simulink model "Smart_City_QCar2_VIRTUAL_car5"  (R2024b)
settings: Solver=ode1  StartTime=0.0  StopTime=inf  FixedStep=Controller_Sample_Time  RelTol=1e-3  EnableMultiTasking=on
values from neighbouring files (symbols this model uses):
  Audio_Sample_Time = 0.3    [Setup_QCar1and2_params.m]
  cameraStepSize = 3e-2    (= 0.03)    [Setup_QCar1and2_params.m]
  CSI_Sample_Time = 1/60    (= 0.0166666666667)    [Setup_QCar1and2_params.m]
  ImageDisplay_Sample_Time = CSI_Sample_Time*6    (= 0.1)    [Setup_QCar1and2_params.m]
  Initialization_Time = 5    [Setup_QCar1and2_params.m]
  LiDAR_Sample_Time = CSI_Sample_Time*3    (= 0.05)    [Setup_QCar1and2_params.m]
  map_mask = [1 1 1 0 0 1 0]    [Setup_QCar1and2_params.m]
  NN_Sample_Time = RealSense_Sample_Time*1    (= 0.0333333333333)    [Setup_QCar1and2_params.m]
  path_x = [0.826 0.836 0.846 0.856 0.866 0.876 0.886 0.896 0.906 0.916 0.926 0.936 ... (740 elements, 740x1)]    [SDCS_Paths_7.mat]
  path_x2 = [-0.614 -0.604 -0.594 -0.584 -0.574 -0.564 -0.554 -0.544 -0.534 -0.524 -0.514 -0.504 ... (1090 elements, 1090x1)]    [SDCS_Paths_7.mat]
  path_x3 = [-0.614 -0.603821428571 -0.593642857143 -0.583464285714 -0.573285714286 -0.563107142857 -0.552928571429 -0.54275 -0.532571428571 -0.522392857143 -0.512214285714 -0.502035714286 ... (714 elements, 714x1)]    [SDCS_Paths_7.mat]
  path_x4 = [-0.614 -0.604 -0.594 -0.584 -0.574 -0.564 -0.554 -0.544 -0.534 -0.524 -0.514 -0.504 ... (1761 elements, 1761x1)]    [SDCS_Paths_7.mat]
  path_x5 = [1.436 1.42588571429 1.41577142857 1.40565714286 1.39554285714 1.38542857143 1.37531428571 1.3652 1.35508571429 1.34497142857 1.33485714286 1.32474285714 ... (574 elements, 574x1)]    [SDCS_Paths_7.mat]
  path_x6 = [1.436 1.42588571429 1.41577142857 1.40565714286 1.39554285714 1.38542857143 1.37531428571 1.3652 1.35508571429 1.34497142857 1.33485714286 1.32474285714 ... (1288 elements, 1288x1)]    [SDCS_Paths_7.mat]
  path_x7 = [-1.5778487585 -1.56959877056 -1.56127865467 -1.55288878259 -1.54442952915 -1.53590127231 -1.52730439309 -1.51863927561 -1.50990630701 -1.50110587746 -1.49223838016 -1.4833042113 ... (2260 elements, 2260x1)]    [SDCS_Paths_7.mat]
  path_y = [-1.0887 -1.0887 -1.0887 -1.0887 -1.0887 -1.0887 -1.0887 -1.0887 -1.0887 -1.0887 -1.0887 -1.0887 ... (740 elements, 740x1)]    [SDCS_Paths_7.mat]
  path_y2 = [-1.0887 -1.0887 -1.0887 -1.0887 -1.0887 -1.0887 -1.0887 -1.0887 -1.0887 -1.0887 -1.0887 -1.0887 ... (1090 elements, 1090x1)]    [SDCS_Paths_7.mat]
  path_y3 = [-1.0887 -1.0887 -1.0887 -1.0887 -1.0887 -1.0887 -1.0887 -1.0887 -1.0887 -1.0887 -1.0887 -1.0887 ... (714 elements, 714x1)]    [SDCS_Paths_7.mat]
  path_y4 = [-1.0887 -1.0887 -1.0887 -1.0887 -1.0887 -1.0887 -1.0887 -1.0887 -1.0887 -1.0887 -1.0887 -1.0887 ... (1761 elements, 1761x1)]    [SDCS_Paths_7.mat]
  path_y5 = [-0.8157 -0.8157 -0.8157 -0.8157 -0.8157 -0.8157 -0.8157 -0.8157 -0.8157 -0.8157 -0.8157 -0.8157 ... (574 elements, 574x1)]    [SDCS_Paths_7.mat]
  path_y6 = [-0.8157 -0.8157 -0.8157 -0.8157 -0.8157 -0.8157 -0.8157 -0.8157 -0.8157 -0.8157 -0.8157 -0.8157 ... (1288 elements, 1288x1)]    [SDCS_Paths_7.mat]
  path_y7 = [-0.614490295955 -0.61974988896 -0.624981792226 -0.630185771997 -0.635361595765 -0.640509032279 -0.645627851559 -0.6507178249 -0.655778724888 -0.660810325409 -0.665812401655 -0.670784730139 ... (2260 elements, 2260x1)]    [SDCS_Paths_7.mat]
  RealSense_Sample_Time = CSI_Sample_Time*2    (= 0.0333333333333)    [Setup_QCar1and2_params.m]
undefined symbols (not defined in the file or in its folder): DiscIntNeverNeededParam, gcbh, Joystick_Sample_Time, JPEG, qc_get_step_size, video_display_show
libraries: quarc_library x61, simulink_extras x9, simulink x5
(part 2 of 4)

== system Smart_City_QCar2_VIRTUAL_car5/Rate Timing Plots/monitorTiming7 ==
  note: Timing Performance
  note: moniorTiming Module:
      |
      | This subsystem outputs the sample time and computation time of the model.
      |
      | Outputs:
      | sampleTime (s) n/a : Sample time (unfiltered and filtered) in seconds.
      | computationTime (s) n/a : Computation time (unfiltered and filtered) in seconds.
      |
      | Usage:
      | Compare the Sample Time (s) output to a constant (qc_get_step_size) to monitor whether or not the desired sample time is being achieved. The Computation Time (s) values should be lower than the corresponding sample time value to ensure that the solver has enough time per time step.
  Computation Time : quarc_library/Sources/Time/Computation Time  sample_time=1  use_model=on  use_cpu_time=off
  Constant : Constant  SampleTime=-1
  Mux : Mux  Inputs=3
  Sample Time : quarc_library/Sources/Time/Sample Time  Priority=-99  sample_time=1
  Timing (s) : Outport  VectorParamsAs1DForOutWhenUnconnected=off
  wires:
  Computation Time/1 -> Mux/3
  Mux/1 -> Timing (s)/1
  Sample Time/1 -> Mux/1
  Constant/1 -> Mux/2

== system Smart_City_QCar2_VIRTUAL_car5/Rate Timing Plots/monitorTiming8 ==
  note: moniorTiming Module:
      |
      | This subsystem outputs the sample time and computation time of the model.
      |
      | Outputs:
      | sampleTime (s) n/a : Sample time (unfiltered and filtered) in seconds.
      | computationTime (s) n/a : Computation time (unfiltered and filtered) in seconds.
      |
      | Usage:
      | Compare the Sample Time (s) output to a constant (qc_get_step_size) to monitor whether or not the desired sample time is being achieved. The Computation Time (s) values should be lower than the corresponding sample time value to ensure that the solver has enough time per time step.
  note: Timing Performance
  Computation Time : quarc_library/Sources/Time/Computation Time  sample_time=Audio_Sample_Time  use_model=on  use_cpu_time=off
  Constant : Constant  Value=Audio_Sample_Time  SampleTime=-1
  Mux : Mux  Inputs=3
  Sample Time : quarc_library/Sources/Time/Sample Time  Priority=-99  sample_time=Audio_Sample_Time
  Timing (s) : Outport  VectorParamsAs1DForOutWhenUnconnected=off
  wires:
  Constant/1 -> Mux/2
  Sample Time/1 -> Mux/1
  Mux/1 -> Timing (s)/1
  Computation Time/1 -> Mux/3

== system Smart_City_QCar2_VIRTUAL_car5/RealSense Camera/Newer Depth ==
  In1 : Inport
  Channel : quarc_library/Signal Routing/Channel  channel=0  buffer_size=1
  Image Compress : quarc_library/Image Processing/Generic/Image Compress  algorithm=JPEG  source=Internal dialog parameter  quality=quality  output_dim=-1
  Video Display : quarc_library/Multimedia/Video Display  Tag=Smart_City_QCar2_VIRTUAL_car5/RealSense Camera/Newer Depth/Video Display  sample_time=sample_time  use_hardware=on
  wires:
  Image Compress/1 -> Channel/1
  In1/1 -> Image Compress/1
  Channel/1 -> Video Display/1

== system Smart_City_QCar2_VIRTUAL_car5/RealSense Camera/obstacleDetection Markham March 22 ==
  note: This function looks within the area of interest and finds the 25% smallest point to use as the distance
  note: m
  note: %
  note: %
  note: px
  note: px
  note: %
  note: m
  note: %
  imageDepth : Inport
  steering (rad) : Inport  Port=2
  new_depth : EnablePort  PropagateVarSize=During execution
  Add : Sum
  Bias : Constant  Value=0
  Box Color : Constant  Value=[255 0 0]
  Constant1 : Constant  Value=200
  Constant2 : Constant  Value=0.1
  Constant3 : Constant  Value=5
  Constant4 : Constant  Value=50
  Constant5 : Constant  Value=.55
  Constant6 : Constant  Value=0.5
  Constant7 : Constant  Value=0.5
  Constant8 : Constant
  Draw Lines Module : MATLAB Function  TreatAsAtomicUnit=on
  Saturation : Saturate  UpperLimit=10  LowerLimit=0.05
  Steering based image subselector : MATLAB Function  TreatAsAtomicUnit=on
  Terminator{,1..6} (7 alike) : Terminator
  imageDepthForDisplay : Outport  VectorParamsAs1DForOutWhenUnconnected=off
  distance (m) : Outport  Port=2
  wires:
  Draw Lines Module/1(img_out) -> imageDepthForDisplay/1
  Box Color/1 -> Draw Lines Module/3(color)
  Constant2/1 -> Steering based image subselector/3(minDistance)
  Constant4/1 -> Steering based image subselector/6(height)
  Steering based image subselector/1(pts) -> Draw Lines Module/2(pts)
  Constant8/1 -> Steering based image subselector/10(maxSteeringWidth)
  Constant7/1 -> Steering based image subselector/9(reduction)
  Constant1/1 -> Steering based image subselector/5(width)
  Constant5/1 -> Steering based image subselector/7(vertCenter)
  Constant6/1 -> Steering based image subselector/8(maxSteering)
  Constant3/1 -> Steering based image subselector/4(maxDistance)
  Saturation/1 -> distance (m)/1
  Bias/1 -> Add/2
  Add/1 -> Saturation/1
  Steering based image subselector/8(pt_25) -> Add/1
  imageDepth/1 -> Steering based image subselector/1(depth), Draw Lines Module/1(img_in)
  steering (rad)/1 -> Steering based image subselector/2(steering)
  Steering based image subselector/2(distance) -> Terminator/1
  Steering based image subselector/3(median_pts) -> Terminator1/1
  Steering based image subselector/4(mean_pts) -> Terminator2/1
  Steering based image subselector/5(min_pts) -> Terminator3/1
  Steering based image subselector/6(max_pts) -> Terminator4/1
  Steering based image subselector/7(num_pts) -> Terminator5/1
  Steering based image subselector/9(mean_middle) -> Terminator6/1

== system Smart_City_QCar2_VIRTUAL_car5/Speed & Steering Commander/Cross Track Controller ==
  closest point : Inport
  distance : Inport  Port=2
  xy : Inport  Port=3
  Heading : Inport  Port=4
  Commanded_Speed : Inport  Port=5
  Path : Inport  Port=6
  Constant : Constant  Value=0
  Constant1 : Constant
  Constant6 : Constant  Value=Initialization_Time
  Cos : Trigonometry  Operator=cos
  Cos1 : Trigonometry
  Cross Product : quarc_library/Math Operations/Vectors/Cross Product
      settings: SourceProductName=QUARC Targets
  Demux : Demux  Outputs=3
  Equal : RelationalOperator  Operator===  OutDataTypeStr=boolean  RndMeth=Simplest  InputSameDT=off
  Equal1 : RelationalOperator  Operator=~=  OutDataTypeStr=boolean  RndMeth=Simplest  InputSameDT=off
  Gain3 : Gain
  Gain6 : Gain  Gain=3
  GreaterThan : RelationalOperator  Operator=<  OutDataTypeStr=boolean  RndMeth=Simplest  InputSameDT=off
  Integrator : Integrator  ExternalReset=level  LimitOutput=on  UpperSaturationLimit=.2  LowerSaturationLimit=-.2
  Integrator1 : Integrator  ExternalReset=level  LimitOutput=on  UpperSaturationLimit=1  LowerSaturationLimit=0
  Memory1 : Memory  InitialCondition=6  InheritSampleTime=on  LinearizeMemory=on  LinearizeAsDelay=on
  Mux : Mux  Inputs=3
  Mux1 : Mux  Inputs=2
  Mux2 : Mux  Inputs=2
  OR : Logic  Operator=OR  Inputs=3  IconShape=distinctive  AllPortsSameDT=off  OutDataTypeStr=boolean
  Product : Product
  Product3 : Product
  Radians to Degrees : simulink_extras/Transformations/Radians to Degrees
  Saturation1 : Saturate  UpperLimit=.2  LowerLimit=-.2
  Scope1 : Scope  NumInputPorts=2
  Sign : Signum
  Sum : Sum  Inputs=+-
  Sum2 : Sum
  Time1 : quarc_library/Sources/Time/Time  time_source=Wall clock  sample_time=qc_get_step_size
  steering correction : Outport
  wires:
  Heading/1 -> Cos1/1, Cos/1
  Cos/1 -> Mux/1
  Cos1/1 -> Mux/2
  xy/1 -> Sum/2
  closest point/1 -> Sum/1
  Sum/1 -> Mux1/1
  Mux1/1 -> Cross Product/2
  Mux/1 -> Cross Product/1
  Cross Product/1 -> Demux/1
  Demux/3 -> Sign/1
  Sign/1 -> Product3/1
  Gain6/1 -> Integrator/1
  Product3/1 -> Gain3/1, Gain6/1
  Integrator/1 -> Mux2/1, Sum2/1
  Saturation1/1 -> Mux2/2, Sum2/2
  distance/1 -> Product3/2
  Sum2/1 -> steering correction/1
  Commanded_Speed/1 -> Equal/1
  Constant/1 -> Equal/2
  Path/1 -> Equal1/2, Memory1/1
  Memory1/1 -> Equal1/1
  Equal1/1 -> OR/2
  Equal/1 -> OR/1
  OR/1 -> Scope1/1, Integrator1/2, Integrator/2
  Constant1/1 -> Integrator1/1
  Product/1 -> Saturation1/1
  Gain3/1 -> Product/1
  Integrator1/1 -> Product/2
  Mux2/1 -> Radians to Degrees/1
  Radians to Degrees/1 -> Scope1/2
  Time1/1 -> GreaterThan/1
  Constant6/1 -> GreaterThan/2
  GreaterThan/1 -> OR/3

== system Smart_City_QCar2_VIRTUAL_car5/Speed & Steering Commander/Infrastructure Car Detection Speed Adjust ==
  obstacleDistance (m) : Inport
  Desired Speed Command : Inport  Port=2
  Constant : Constant  Value=0.3
  Constant1 : Constant  Value=.4
  Constant2 : Constant
  Less Than : RelationalOperator  Operator=<  OutDataTypeStr=boolean  RndMeth=Simplest  InputSameDT=off
  MATLAB Function : MATLAB Function  TreatAsAtomicUnit=on
  Scope : Scope  NumInputPorts=2
  Adjusted Speed Command : Outport  VectorParamsAs1DForOutWhenUnconnected=off
  Honk : Outport  Port=2
  wires:
  Desired Speed Command/1 -> MATLAB Function/4(nominal_speed)
  MATLAB Function/1(speed_cmd) -> Adjusted Speed Command/1, Scope/1
  Less Than/1 -> Honk/1
  Constant1/1 -> Less Than/2
  obstacleDistance (m)/1 -> MATLAB Function/1(obstacle_distance), Scope/2, Less Than/1
  Constant/1 -> MATLAB Function/2(stop_distance)  "stop distance (m)"
  Constant2/1 -> MATLAB Function/3(nominal_tracking_distance)  "nominal tracking distance (m)"

== system Smart_City_QCar2_VIRTUAL_car5/Speed & Steering Commander/Path Commander ==
  note: Tunable
      | Params
  note: Changed the abs and the duration
  path : Inport
  xy : Inport  Port=2
  look_ahead_d : Inport  Port=3
  Data Type Conversion : DataTypeConversion  SaturateOnIntegerOverflow=off  RndMeth=Floor
  Display : Display
  "Distance  " : Scope
  Distance (m) to a viable path : Constant  Value=0.05
  Duration that car is within distance of viable path : Constant  Value=0.35
  Less Than Threshold : Subsystem
  Multiport Switch : MultiPortSwitch  Inputs=7  DiagnosticForDefault=None  SaturateOnIntegerOverflow=off  InputSameDT=off
  Multiport Switch1 : MultiPortSwitch  Inputs=7  DiagnosticForDefault=None  SaturateOnIntegerOverflow=off  InputSameDT=off
  Multiport Switch2 : MultiPortSwitch  Inputs=7  DiagnosticForDefault=None  SaturateOnIntegerOverflow=off  InputSameDT=off
  Mux : Mux  Inputs=7
  Path 1  Look Ahead Generator : Subsystem
  Path 2  Look Ahead Generator : Subsystem
  Path 3  Look Ahead Generator : Subsystem
  Path 4  Look Ahead Generator : Subsystem
  Path 5  Look Ahead Generator : Subsystem
  Path 6  Look Ahead Generator : Subsystem
  Path 7  Look Ahead Generator : Subsystem
  Turn Paths on and Off : Gain  Gain=map_mask
  xy_cmd : Outport
  Path_Options : Outport  Port=2
  closest point : Outport  Port=3
  distance : Outport  Port=4
  wires:
  look_ahead_d/1 -> Path 7  Look Ahead Generator/2(look_ahead_d), Path 6  Look Ahead Generator/2(look_ahead_d), Path 5  Look Ahead Generator/2(look_ahead_d), Path 4  Look Ahead Generator/2(look_ahead_d), Path 3  Look Ahead Generator/2(look_ahead_d), Path 2  Look Ahead Generator/2(look_ahead_d), Path 1  Look Ahead Generator/2(look_ahead_d)
  path/1 -> Multiport Switch2/1, Multiport Switch1/1, Multiport Switch/1
  Path 1  Look Ahead Generator/1(xy_cmd) -> Multiport Switch/2
  Path 2  Look Ahead Generator/1(xy_cmd) -> Multiport Switch/3
  Multiport Switch/1 -> xy_cmd/1
  Path 3  Look Ahead Generator/1(xy_cmd) -> Multiport Switch/4
  Path 4  Look Ahead Generator/1(xy_cmd) -> Multiport Switch/5
  Path 1  Look Ahead Generator/3(distance) -> Multiport Switch2/2, Mux/1
  Path 2  Look Ahead Generator/3(distance) -> Multiport Switch2/3, Mux/2
  Path 3  Look Ahead Generator/3(distance) -> Multiport Switch2/4, Mux/3
  Path 4  Look Ahead Generator/3(distance) -> Multiport Switch2/5, Mux/4
  Mux/1 -> "Distance  "/1, Less Than Threshold/1(Distances)
  Distance (m) to a viable path/1 -> Less Than Threshold/2(Distance Threshold)
  Duration that car is within distance of viable path/1 -> Less Than Threshold/3(Duration Threshold)
  Less Than Threshold/1(elapsed) -> Data Type Conversion/1, Display/1
  Turn Paths on and Off/1 -> Path_Options/1
  Data Type Conversion/1 -> Turn Paths on and Off/1
  Path 5  Look Ahead Generator/1(xy_cmd) -> Multiport Switch/6
  Path 6  Look Ahead Generator/1(xy_cmd) -> Multiport Switch/7
  Path 5  Look Ahead Generator/3(distance) -> Multiport Switch2/6, Mux/5
  Path 6  Look Ahead Generator/3(distance) -> Multiport Switch2/7, Mux/6
  Path 1  Look Ahead Generator/2(closest_point) -> Multiport Switch1/2
  Path 2  Look Ahead Generator/2(closest_point) -> Multiport Switch1/3
  Path 3  Look Ahead Generator/2(closest_point) -> Multiport Switch1/4
  Path 4  Look Ahead Generator/2(closest_point) -> Multiport Switch1/5
  Path 5  Look Ahead Generator/2(closest_point) -> Multiport Switch1/6
  Path 6  Look Ahead Generator/2(closest_point) -> Multiport Switch1/7
  Multiport Switch1/1 -> closest point/1
  Multiport Switch2/1 -> distance/1
  xy/1 -> Path 7  Look Ahead Generator/1(xy), Path 6  Look Ahead Generator/1(xy), Path 5  Look Ahead Generator/1(xy), Path 4  Look Ahead Generator/1(xy), Path 3  Look Ahead Generator/1(xy), Path 2  Look Ahead Generator/1(xy), Path 1  Look Ahead Generator/1(xy)
  Path 7  Look Ahead Generator/1(xy_cmd) -> Multiport Switch/8
  Path 7  Look Ahead Generator/2(closest_point) -> Multiport Switch1/8
  Path 7  Look Ahead Generator/3(distance) -> Mux/7, Multiport Switch2/8

== system Smart_City_QCar2_VIRTUAL_car5/Speed & Steering Commander/Realsense Obstacle Detection Speed Adjust ==
  obstacleDistance (m) : Inport
  Desired Speed Command : Inport  Port=2
  Constant : Constant  Value=0.5
  Constant1 : Constant  Value=0.5
  Constant2 : Constant  Value=0.75
  Less Than : RelationalOperator  Operator=<  OutDataTypeStr=boolean  RndMeth=Simplest  InputSameDT=off
  MATLAB Function : MATLAB Function  TreatAsAtomicUnit=on
  Scope : Scope  NumInputPorts=2
  Adjusted Speed Command : Outport  VectorParamsAs1DForOutWhenUnconnected=off
  Honk : Outport  Port=2
  wires:
  Constant2/1 -> MATLAB Function/3(nominal_tracking_distance)  "nominal tracking distance (m)"
  Constant/1 -> MATLAB Function/2(stop_distance)  "stop distance (m)"
  obstacleDistance (m)/1 -> Less Than/1, Scope/2, MATLAB Function/1(obstacle_distance)
  Constant1/1 -> Less Than/2
  Less Than/1 -> Honk/1
  MATLAB Function/1(speed_cmd) -> Scope/1, Adjusted Speed Command/1
  Desired Speed Command/1 -> MATLAB Function/4(nominal_speed)

== system Smart_City_QCar2_VIRTUAL_car5/Speed & Steering Commander/Steering Based on LiDAR ==
  xy_command : Inport
  xy : Inport  Port=2
  heading : Inport  Port=3
  Direction Vector Generator : Subsystem
  Display1 : Display
      settings: Decimation=100
  Gain1 : Gain
  Radians to Degrees1 : simulink_extras/Transformations/Radians to Degrees
  Steering Commander : MATLAB Function  TreatAsAtomicUnit=on
  distance : Outport
  LiDAR Steering : Outport  Port=2
  wires:
  Direction Vector Generator/1(distance) -> distance/1
  xy_command/1 -> Direction Vector Generator/1(xy_command)
  Direction Vector Generator/2(aoa) -> Radians to Degrees1/1, Steering Commander/1(aoa)
  Gain1/1 -> LiDAR Steering/1
  Radians to Degrees1/1 -> Display1/1
  xy/1 -> Direction Vector Generator/2(xy)
  heading/1 -> Direction Vector Generator/3(heading)
  Steering Commander/1(steering) -> Gain1/1

== system Smart_City_QCar2_VIRTUAL_car5/Speed & Steering Commander/Traffic Zone 1 ==
  note: [1 -.3] %[1,5 0]
  note: [0.2 -0.7]
  note: select the control variable
  xy : Inport
  speed in : Inport  Port=2
  Traffic Light : Inport  Port=3
  AND : Logic  Inputs=4  IconShape=distinctive  AllPortsSameDT=off  OutDataTypeStr=boolean
  Bias : Bias  SaturateOnIntegerOverflow=off
  Constant13 : Constant  Value=[-0.61 -1.21]
  Constant14 : Constant  Value=[0 -0.86]
  Constant3 : Constant  Value=.1
  Demux : Demux  Outputs=2
  Demux1 : Demux  Outputs=2
  Demux2 : Demux  Outputs=2
  Display : Display
  Gain : Gain  Gain=-1
  Greater Than Threshold : Subsystem
  Less Than Threshold : Subsystem
  MATLAB Function2 : MATLAB Function  TreatAsAtomicUnit=on
  Memory7 : Memory  InitialCondition=1  InheritSampleTime=on  LinearizeMemory=on  LinearizeAsDelay=on
  Saturation : Saturate  UpperLimit=1  LowerLimit=0
  "Speed " : Scope
  Speed Multi : Scope
  Traffic State : Display
  in zone : Display
  Speed Out : Outport
  wires:
  xy/1 -> Greater Than Threshold/1(Signal), Less Than Threshold/1(Signal), Demux2/1
  Constant3/1 -> Less Than Threshold/3(Duration), Greater Than Threshold/3(Duration)
  Constant13/1 -> Greater Than Threshold/2(Threshold)
  Constant14/1 -> Less Than Threshold/2(Threshold)
  Greater Than Threshold/1(elapsed) -> Demux/1
  Demux/2 -> AND/2
  Demux/1 -> AND/1
  Less Than Threshold/1(elapsed) -> Demux1/1
  Demux1/2 -> AND/4
  Demux1/1 -> AND/3
  Demux2/1 -> Bias/1
  Bias/1 -> Gain/1
  Gain/1 -> Saturation/1
  MATLAB Function2/1(Traffic_State) -> Memory7/1, Traffic State/1
  Memory7/1 -> MATLAB Function2/1(Previous_State)
  speed in/1 -> MATLAB Function2/2(Speed_In)
  AND/1 -> MATLAB Function2/4(In_Zone), in zone/1
  Saturation/1 -> Speed Multi/1, MATLAB Function2/3(Speed_Multi)
  MATLAB Function2/2(Speed_Out) -> Speed Out/1, "Speed "/1
  Traffic Light/1 -> Display/1, MATLAB Function2/5(Traffic_Light)  "1 means green"

== system Smart_City_QCar2_VIRTUAL_car5/Speed & Steering Commander/Traffic Zone 2 ==
  note: select the control variable
  xy : Inport
  speed in : Inport  Port=2
  Traffic Light : Inport  Port=3
  AND : Logic  Inputs=4  IconShape=distinctive  AllPortsSameDT=off  OutDataTypeStr=boolean
  Bias : Bias  Bias=-0.8  SaturateOnIntegerOverflow=off
  Constant13 : Constant  Value=[0.75 -0.9]
  Constant14 : Constant  Value=[1.35 -0.65]
  Constant3 : Constant  Value=.1
  Demux : Demux  Outputs=2
  Demux1 : Demux  Outputs=2
  Demux2 : Demux  Outputs=2
  Display : Display
  Gain : Gain
  Greater Than Threshold : Subsystem
  Less Than Threshold : Subsystem
  MATLAB Function2 : MATLAB Function  TreatAsAtomicUnit=on
  Memory7 : Memory  InitialCondition=1  InheritSampleTime=on  LinearizeMemory=on  LinearizeAsDelay=on
  Saturation : Saturate  UpperLimit=1  LowerLimit=0
  "Speed " : Scope
  Speed Multi : Scope
  Traffic State : Display
  in zone : Display
  Speed Out : Outport
  wires:
  MATLAB Function2/2(Speed_Out) -> "Speed "/1, Speed Out/1
  Saturation/1 -> MATLAB Function2/3(Speed_Multi), Speed Multi/1
  AND/1 -> in zone/1, MATLAB Function2/4(In_Zone)
  speed in/1 -> MATLAB Function2/2(Speed_In)
  Memory7/1 -> MATLAB Function2/1(Previous_State)
  MATLAB Function2/1(Traffic_State) -> Traffic State/1, Memory7/1
  Gain/1 -> Saturation/1
  Bias/1 -> Gain/1
  Demux2/1 -> Bias/1
  Demux1/1 -> AND/3
  Demux1/2 -> AND/4
  Less Than Threshold/1(elapsed) -> Demux1/1
  Demux/1 -> AND/1
  Demux/2 -> AND/2
  Greater Than Threshold/1(elapsed) -> Demux/1
  Constant14/1 -> Less Than Threshold/2(Threshold)
  Constant13/1 -> Greater Than Threshold/2(Threshold)
  Constant3/1 -> Greater Than Threshold/3(Duration), Less Than Threshold/3(Duration)
  xy/1 -> Greater Than Threshold/1(Signal), Less Than Threshold/1(Signal), Demux2/1
  Traffic Light/1 -> Display/1, MATLAB Function2/5(Traffic_Light)

== system Smart_City_QCar2_VIRTUAL_car5/Speed & Steering Commander/xy signal maker ==
  xy 1 : Inport
  xy 2 : Inport  Port=2
  Demux1 : Demux  Outputs=2
  Demux2 : Demux  Outputs=2
  Mux : Mux  Inputs=2
  Mux1 : Mux  Inputs=2
  Rate Transition1 : RateTransition  OutPortSampleTime=ImageDisplay_Sample_Time
  Rate Transition2 : RateTransition  OutPortSampleTime=ImageDisplay_Sample_Time
  x : Outport
  y : Outport  Port=2
  wires:
  Demux2/1 -> Mux/2
  Demux1/2 -> Mux1/1
  Demux1/1 -> Mux/1
  Demux2/2 -> Mux1/2
  Mux/1 -> x/1
  Mux1/1 -> y/1
  xy 1/1 -> Rate Transition1/1
  Rate Transition1/1 -> Demux1/1
  xy 2/1 -> Rate Transition2/1
  Rate Transition2/1 -> Demux2/1

== system Smart_City_QCar2_VIRTUAL_car5/QCar/To//From Simulation/RGB ==
  In1 : Inport
  Enable : EnablePort  StatesWhenEnabling=reset
  Image Decompress : quarc_library/Image Processing/Generic/Image Decompress  algorithm=JPEG  resolution=custom  width=820  height=410  output_format=MATLAB RGB (HxWx3)  data_type=uint8
      settings: AttributesFormatString=(%<algorithm>)  SourceProductName=QUARC Targets
  RGB : Outport  VectorParamsAs1DForOutWhenUnconnected=off
  wires:
  Image Decompress/1 -> RGB/1
  In1/1 -> Image Decompress/1

== system Smart_City_QCar2_VIRTUAL_car5/QCar/To//From Simulation/RGB1 ==
  In1 : Inport
  Enable : EnablePort  StatesWhenEnabling=reset
  Image Decompress : quarc_library/Image Processing/Generic/Image Decompress  algorithm=JPEG  resolution=custom  width=820  height=410  output_format=MATLAB RGB (HxWx3)  data_type=uint8
      settings: AttributesFormatString=(%<algorithm>)  SourceProductName=QUARC Targets
  RGB : Outport  VectorParamsAs1DForOutWhenUnconnected=off
  wires:
  Image Decompress/1 -> RGB/1
  In1/1 -> Image Decompress/1

== system Smart_City_QCar2_VIRTUAL_car5/QCar/To//From Simulation/RGB2 ==
  In1 : Inport
  Enable : EnablePort  StatesWhenEnabling=reset
  Image Decompress : quarc_library/Image Processing/Generic/Image Decompress  algorithm=JPEG  resolution=custom  width=820  height=410  output_format=MATLAB RGB (HxWx3)  data_type=uint8
      settings: AttributesFormatString=(%<algorithm>)  SourceProductName=QUARC Targets
  RGB : Outport  VectorParamsAs1DForOutWhenUnconnected=off
  wires:
  Image Decompress/1 -> RGB/1
  In1/1 -> Image Decompress/1

== system Smart_City_QCar2_VIRTUAL_car5/QCar/To//From Simulation/RGB3 ==
  In1 : Inport
  Enable : EnablePort  StatesWhenEnabling=reset
  Image Decompress : quarc_library/Image Processing/Generic/Image Decompress  algorithm=JPEG  resolution=custom  width=820  height=410  output_format=MATLAB RGB (HxWx3)  data_type=uint8
      settings: AttributesFormatString=(%<algorithm>)  SourceProductName=QUARC Targets
  RGB : Outport  VectorParamsAs1DForOutWhenUnconnected=off
  wires:
  Image Decompress/1 -> RGB/1
  In1/1 -> Image Decompress/1

== system Smart_City_QCar2_VIRTUAL_car5/QCar/To//From Simulation/RGB4 ==
  In1 : Inport
  Enable : EnablePort  StatesWhenEnabling=reset
  Image Decompress : quarc_library/Image Processing/Generic/Image Decompress  algorithm=JPEG  resolution=640 x 480  width=640  height=480  output_format=MATLAB RGB (HxWx3)  data_type=uint8
      settings: AttributesFormatString=(%<algorithm>)  SourceProductName=QUARC Targets
  RGB : Outport  VectorParamsAs1DForOutWhenUnconnected=off
  wires:
  Image Decompress/1 -> RGB/1
  In1/1 -> Image Decompress/1

== system Smart_City_QCar2_VIRTUAL_car5/QCar/To//From Simulation/RGB5 ==
  In1 : Inport
  Enable : EnablePort  StatesWhenEnabling=reset
  Image Decompress : quarc_library/Image Processing/Generic/Image Decompress  algorithm=JPEG  resolution=640 x 480  width=640  height=480  output_format=MATLAB greyscale (HxW)  data_type=uint8
      settings: AttributesFormatString=(%<algorithm>)  SourceProductName=QUARC Targets
  RGB : Outport  VectorParamsAs1DForOutWhenUnconnected=off
  wires:
  Image Decompress/1 -> RGB/1
  In1/1 -> Image Decompress/1

== system Smart_City_QCar2_VIRTUAL_car5/QCar/To//From Simulation/Subsystem ==
  dist : Inport
  angles : Inport  Port=2
  Gain : Gain  Gain=0.1
  Polar Figure : quarc_library/Sinks/Figures/Polar Figure  figure_mode=Use figure window  figure_tag=figure1  axes_tag=axes1  plot_mode=Frame-based  minimum_rho=0  maximum_rho=2  minimum_theta=0  maximum_theta=360  zero_location=top  direction=counterclockwise  buffer_size=1  update_rate=100  sample_time=-1  initial_position="2561      343.66667           1920      983.33333"  initial_visibility=off  line1_style=Solid line (-)  line1_width=0.5  line1_color=[0 0.4470 0.7410]  marker1=Circle (o)  marker1_size=2  marker1_edge_color=[0 0.447059 0.741176]  marker1_face_color=[0 0.447059 0.741176]  line2_style=Solid line (-)  line2_width=0.5  line2_color=[0.85098 0.32549 0.0980392]  marker2=None  marker2_size=6  marker2_edge_color=[0.85098 0.32549 0.0980392]  marker2_face_color=[0.85098 0.32549 0.0980392]  line3_style=Solid line (-)  line3_width=0.5  line3_color=[0.929412 0.694118 0.12549]  marker3=None  marker3_size=6  marker3_edge_color=[0.929412 0.694118 0.12549]  marker3_face_color=[0.929412 0.694118 0.12549]  line4_style=Solid line (-)  line4_width=0.5  line4_color=[0.494118 0.184314 0.556863]  marker4=None  marker4_size=6  marker4_edge_color=[0.494118 0.184314 0.556863]  marker4_face_color=[0.494118 0.184314 0.556863]  line5_style=Solid line (-)  line5_width=0.5  line5_color=[0.466667 0.67451 0.188235]  marker5=None  marker5_size=6  marker5_edge_color=[0.466667 0.67451 0.188235]  marker5_face_color=[0.466667 0.67451 0.188235]
      settings: SourceProductName=QUARC Targets
  wires:
  Gain/1 -> Polar Figure/1
  dist/1 -> Gain/1
  angles/1 -> Polar Figure/2

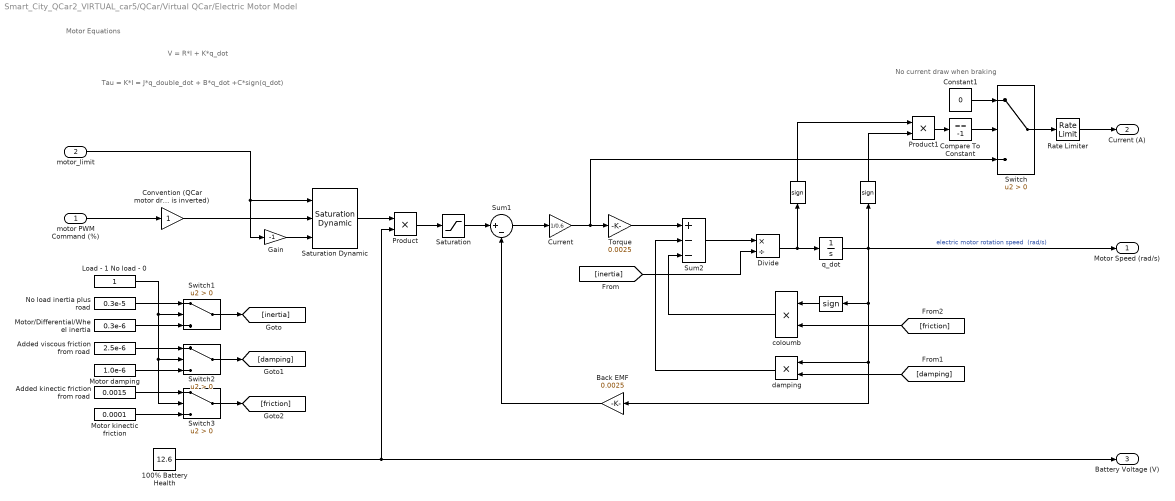
== system Smart_City_QCar2_VIRTUAL_car5/QCar/Virtual QCar/Electric Motor Model ==
  note: No current draw when braking
  note: Motor Equations
  note: Tau = K*I = J*q_double_dot + B*q_dot +C*sign(q_dot)
  note: V = R*I + K*q_dot
  motor PWM Command (%) : Inport
  motor_limit : Inport  Port=2
  " " : Signum
  "  " : Signum
  "   " : Signum
  100% Battery Health : Constant  Value=12.6
  Added kinectic friction from road : Constant  Value=0.0015
  Added viscous friction from road : Constant  Value=2.5e-6
  Back EMF : Gain  Gain=0.0025
  Compare To Constant : simulink/Logic and Bit Operations/Compare To Constant  relop===  const=-1  OutDataTypeStr=boolean
  Constant1 : Constant  Value=0
  Convention (QCar motor drive is inverted) : Gain
  Current : Gain  Gain=1/0.6
  Divide : Product  Inputs=*/
  Gain : Gain  Gain=-1
  Load - 1 No load - 0 : Constant
  Motor damping : Constant  Value=1.0e-6
  Motor kinectic friction : Constant  Value=0.0001
  Motor/Differential/Wheel inertia : Constant  Value=0.3e-6
  No load inertia plus road : Constant  Value=0.3e-5
  Product : Product
  Product1 : Product
  Rate Limiter : RateLimiter  RisingSlewLimit=1*10  FallingSlewLimit=-1*10  SampleTimeMode=inherited
  Saturation : Saturate  UpperLimit=12.6  LowerLimit=-12.6
  Saturation Dynamic : simulink/Discontinuities/Saturation Dynamic  OutMin=[]  OutMax=[]  OutDataTypeStr=Inherit: Same as second input  OutDataType=fixdt(1, 16)  OutScaling=2^-10  DoSatur=off
  Sum1 : Sum  Inputs=|+-
  Sum2 : Sum  Inputs=+--
  Switch{,1..3} (4 alike) : Switch  Criteria=u2 > Threshold  SaturateOnIntegerOverflow=off  InputSameDT=off
  Torque : Gain  Gain=0.0025
  coloumb : Product
  damping : Product
  q_dot : Integrator
  Motor Speed (rad/s) : Outport
  Current (A) : Outport  Port=2
  Battery Voltage (V) : Outport  Port=3
  wires:
  Back EMF/1 -> Sum1/2
  q_dot/1 -> "  "/1, " "/1, Back EMF/1, damping/1, Motor Speed (rad/s)/1  "electric motor rotation speed  (rad/s)"
  coloumb/1 -> Sum2/3
  Sum1/1 -> Current/1
  100% Battery Health/1 -> Product/2, Battery Voltage (V)/1
  Sum2/1 -> Divide/1
  Torque/1 -> Sum2/1
  "  "/1 -> Product1/2
  damping/1 -> Sum2/2
  Divide/1 -> q_dot/1, "   "/1
  Product/1 -> Saturation/1
  motor PWM Command (%)/1 -> Convention (QCar motor drive is inverted)/1
  Saturation Dynamic/1 -> Product/1
  motor_limit/1 -> Gain/1, Saturation Dynamic/1
  Gain/1 -> Saturation Dynamic/3
  Convention (QCar motor drive is inverted)/1 -> Saturation Dynamic/2
  [damping] -> damping/2
  [friction] -> coloumb/2
  Current/1 -> Torque/1, Switch/3
  Saturation/1 -> Sum1/1
  "   "/1 -> Product1/1
  Product1/1 -> Compare To Constant/1
  Compare To Constant/1 -> Switch/2
  Constant1/1 -> Switch/1
  Switch/1 -> Rate Limiter/1
  Rate Limiter/1 -> Current (A)/1
  Load - 1 No load - 0/1 -> Switch2/2, Switch3/2, Switch1/2
  No load inertia plus road/1 -> Switch1/1
  Motor/Differential/Wheel inertia/1 -> Switch1/3
  Added viscous friction from road/1 -> Switch2/1
  Motor damping/1 -> Switch2/3
  Added kinectic friction from road/1 -> Switch3/1
  Motor kinectic friction/1 -> Switch3/3
  Switch1/1 -> [inertia]
  Switch2/1 -> [damping]
  Switch3/1 -> [friction]
  [inertia] -> Divide/2
  " "/1 -> coloumb/1

== system Smart_City_QCar2_VIRTUAL_car5/QCar/Virtual QCar/LED Logic ==
  note: Headlights, Brakes, Left, Right
  Speed : Inport
  Throttle : Inport  Port=2
  Steering : Inport  Port=3
  Headlights : Inport  Port=4
  " Brake" : Logic  Operator=OR  IconShape=distinctive  AllPortsSameDT=off  OutDataTypeStr=boolean
  AND : Logic  IconShape=distinctive  AllPortsSameDT=off  OutDataTypeStr=boolean
  Constant1 : Constant  Value=20
  Constant2 : Constant  Value=.1
  Constant3 : Constant  Value=0
  Constant4 : Constant  Value=.1
  Constant5 : Constant  Value=0
  Constant6 : Constant  Value=.2
  Constant7 : Constant  Value=.01
  Constant8 : Constant  Value=.1
  Gain : Gain  Gain=-1
  Gain1 : Gain  Gain=-1
  Greater Than Threshold1 : Subsystem
  Left Threshold : Subsystem
  Less Than Threshold1 : Subsystem
  Less Than Threshold2 : Subsystem
  Less Than Threshold3 : Subsystem
  MATLAB Function : MATLAB Function  TreatAsAtomicUnit=on
  Pulse Generator : DiscretePulseGenerator  Period=500  PulseWidth=250  SampleTime=qc_get_step_size
  Radians to Degrees : simulink_extras/Transformations/Radians to Degrees
  Right Threshold : Subsystem
  LEDs : Outport
  wires:
  Gain1/1 -> Greater Than Threshold1/2(Threshold)
  AND/1 -> " Brake"/2
  Greater Than Threshold1/1(elapsed) -> AND/2
  Less Than Threshold3/1(elapsed) -> AND/1
  Constant8/1 -> Less Than Threshold3/2(Threshold), Gain1/1
  Constant7/1 -> Greater Than Threshold1/3(Duration), Less Than Threshold3/3(Duration)
  Less Than Threshold2/1(elapsed) -> " Brake"/1
  Constant6/1 -> Less Than Threshold2/3(Duration)
  Constant5/1 -> Less Than Threshold2/2(Threshold)
  Throttle/1 -> Less Than Threshold2/1(Signal)
  Constant4/1 -> Less Than Threshold1/3(Duration)
  Constant3/1 -> Less Than Threshold1/2(Threshold)
  Speed/1 -> Less Than Threshold1/1(Signal), Greater Than Threshold1/1(Signal), Less Than Threshold3/1(Signal)
  Gain/1 -> Right Threshold/2(Threshold)
  Constant2/1 -> Left Threshold/3(Duration), Right Threshold/3(Duration)
  Constant1/1 -> Left Threshold/2(Threshold), Gain/1
  Radians to Degrees/1 -> Left Threshold/1(Signal), Right Threshold/1(Signal)
  Steering/1 -> Radians to Degrees/1
  MATLAB Function/1(lights) -> LEDs/1
  Pulse Generator/1 -> MATLAB Function/6(pulse)
  Headlights/1 -> MATLAB Function/1(headlights)
  " Brake"/1 -> MATLAB Function/2(breaklights)
  Left Threshold/1(elapsed) -> MATLAB Function/4(leftTurn)
  Right Threshold/1(elapsed) -> MATLAB Function/5(rightTurn)

== system Smart_City_QCar2_VIRTUAL_car5/QCar/Virtual QCar/basicSpeedEstimation ==
  note: Estimate car speed from motor encoder counts rate
  note: v = 2*pi*r * omega (if omega is in rot/s)
      | v = r * omega (if omega is in rad/s)
      | r = 0.0342 m
  note: (Diff. pinion*pinion)/(Spur*Diff. spur)
  note: speedEstimation Module:
      |
      | This subsystem converts the motor speed measurements in counts/s to a useful longitudinal car speed in m/s.
      |
      | Inputs:
      | motorSpeed (counts/s) n/a : Drive motor speed measured using an encoder
      |
      | Outputs:
      | longitudinalCarSpeed (m/s) n/a : The platform's longitudinal speed (along the front-rear axis direction)
  motorSpeed (rad/s) : Inport
  gear ratios : Gain  Gain=(13*19)/(70*37)
  to rot/s : Gain
  wheel radius : Gain  Gain=0.0342
  longitudinalCarSpeed (m/s) : Outport  VectorParamsAs1DForOutWhenUnconnected=off
  wires:
  motorSpeed (rad/s)/1 -> to rot/s/1  "motor speed (rot/s)"
  wheel radius/1 -> longitudinalCarSpeed (m/s)/1  "wheel speed (m/s)"
  gear ratios/1 -> wheel radius/1  "shaft speed (rots/s)"
  to rot/s/1 -> gear ratios/1  "wheel speed (m/s)"

== system Smart_City_QCar2_VIRTUAL_car5/QCar/Virtual QCar/speedController ==
  note: Feedforward
  note: Feedback
  arm (0,1) : Inport
  desiredSpeed (m/s) : Inport  Port=2
  measuredSpeed (m/s) : Inport  Port=3
  Add : Sum
  Add1 : Sum
  Compare To Zero : simulink/Logic and Bit Operations/Compare To Zero  relop===  OutDataTypeStr=boolean
  Integrator1 : Integrator  ExternalReset=either  LimitOutput=on  UpperSaturationLimit=0.4  LowerSaturationLimit=-0.4
  Kff (% / m/s) : Gain  Gain=0.1
  "Ki (% / m) " : Gain  Gain=.5
  Kp (% / m/s) : Gain  Gain=.5
  Multiply : Product
  Multiply1 : Product
  Multiply2 : Product
  Speed_Tracking : Scope  NumInputPorts=2
  Sum : Sum  Inputs=|+-
  command saturation : Saturate  UpperLimit=5  LowerLimit=-5
  PWM Cmd : Outport  VectorParamsAs1DForOutWhenUnconnected=off
  wires:
  command saturation/1 -> Multiply1/1  "desired"
  arm (0,1)/1 -> Multiply1/2, Multiply/2, Multiply2/2
  measuredSpeed (m/s)/1 -> Multiply/1  "meas"
  Multiply/1 -> Sum/2, Speed_Tracking/2  "measured"
  Add/1 -> Add1/2
  Add1/1 -> Multiply2/1  "%"
  Multiply1/1 -> Compare To Zero/1, Sum/1, Kff (% / m/s)/1, Speed_Tracking/1  "desired"
  Integrator1/1 -> Add/2
  Kp (% / m/s)/1 -> Add/1
  Compare To Zero/1 -> Integrator1/2
  Kff (% / m/s)/1 -> Add1/1
  Sum/1 -> "Ki (% / m) "/1, Kp (% / m/s)/1
  "Ki (% / m) "/1 -> Integrator1/1
  Multiply2/1 -> PWM Cmd/1  "pwm duty cycle"
  desiredSpeed (m/s)/1 -> command saturation/1

== system Smart_City_QCar2_VIRTUAL_car5/Randomizer1/Subsystem1/RisingEdge ==
  Input : Inport
  Logical Operator1 : Logic  AllPortsSameDT=off
  Logical Operator2 : Logic  Operator=NOT  AllPortsSameDT=off
  Memory : Memory  InheritSampleTime=on  LinearizeMemory=on
  RisingEdgeTrigger : Outport  VectorParamsAs1DForOutWhenUnconnected=off
  wires:
  Logical Operator1/1 -> RisingEdgeTrigger/1
  Logical Operator2/1 -> Logical Operator1/2
  Memory/1 -> Logical Operator2/1
  Input/1 -> Logical Operator1/1, Memory/1

== system Smart_City_QCar2_VIRTUAL_car5/Speed & Steering Commander/Path Commander/Less Than Threshold ==
  note: Calculate Duration that Car is in Distance of Viable Path
  Distances : Inport
  Distance Threshold : Inport  Port=2
  Duration Threshold : Inport  Port=3
  Data Type Conversion : DataTypeConversion  SaturateOnIntegerOverflow=off  RndMeth=Floor
  Discrete-Time Integrator : DiscreteIntegrator  Priority=1  ExternalReset=level  SampleTime=qc_get_step_size  ICPrevOutput=DiscIntNeverNeededParam  ICPrevScaledInput=DiscIntNeverNeededParam
  Relational Operator : RelationalOperator  Operator=<  InputSameDT=off
  Relational Operator1 : RelationalOperator  InputSameDT=off
  Reset Condition : Logic  Operator=NOT  AllPortsSameDT=off  OutDataTypeStr=boolean
  elapsed : Outport  VectorParamsAs1DForOutWhenUnconnected=off
  wires:
  Data Type Conversion/1 -> Discrete-Time Integrator/1
  Distances/1 -> Relational Operator/1
  Distance Threshold/1 -> Relational Operator/2
  Relational Operator/1 -> Data Type Conversion/1, Reset Condition/1
  Reset Condition/1 -> Discrete-Time Integrator/2
  Discrete-Time Integrator/1 -> Relational Operator1/1
  Duration Threshold/1 -> Relational Operator1/2
  Relational Operator1/1 -> elapsed/1

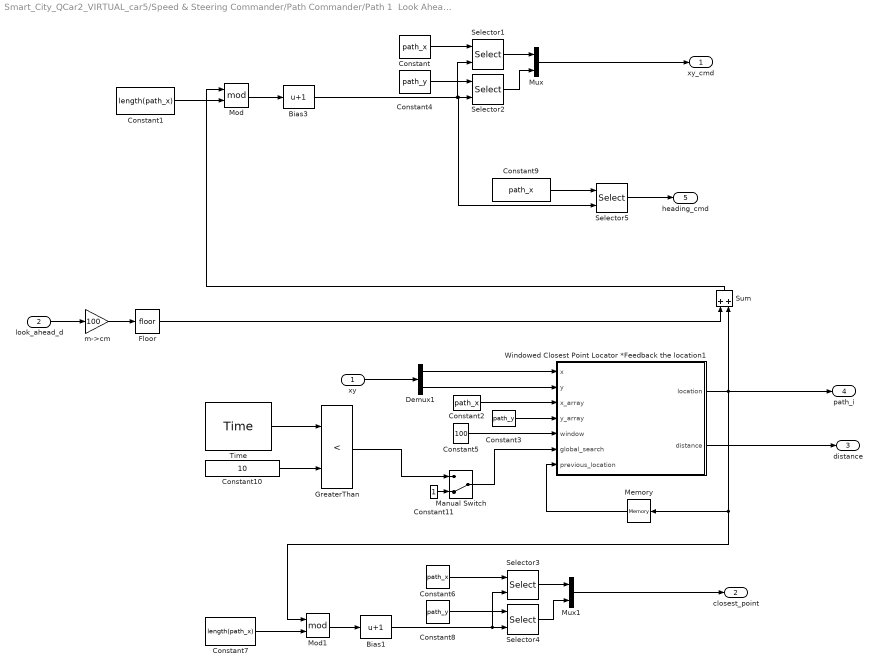
== system Smart_City_QCar2_VIRTUAL_car5/Speed & Steering Commander/Path Commander/Path 1  Look Ahead Generator ==
  xy : Inport
  look_ahead_d : Inport  Port=2
  Bias1 : Bias  Bias=1  SaturateOnIntegerOverflow=off
  Bias3 : Bias  Bias=1  SaturateOnIntegerOverflow=off
  Constant{,2,6,9} (4 alike) : Constant  Value=path_x
  Constant1 : Constant  Value=length(path_x)
  Constant10 : Constant  Value=10
  Constant11 : Constant
  Constant3 : Constant  Value=path_y
  Constant4 : Constant  Value=path_y
  Constant5 : Constant  Value=100
  Constant7 : Constant  Value=length(path_x)
  Constant8 : Constant  Value=path_y
  Demux1 : Demux  Outputs=2
  Floor : Rounding
  GreaterThan : RelationalOperator  Operator=<  OutDataTypeStr=boolean  RndMeth=Simplest  InputSameDT=off
  Manual Switch : ManualSwitch  CurrentSetting=0
  Memory : Memory  InitialCondition=1  InheritSampleTime=on  LinearizeMemory=on  LinearizeAsDelay=on
  Mod : Math  Operator=mod
  Mod1 : Math  Operator=mod
  Mux : Mux  Inputs=2
  Mux1 : Mux  Inputs=2
  Selector{1..5} (5 alike) : Selector  InputPortWidth=length(path_x)  IndexOptions=Index vector (port)  Indices=[1 3]  OutputSizes=1
  Sum : Sum
  Time : quarc_library/Sources/Time/Time  time_source=Wall clock  sample_time=qc_get_step_size
  Windowed Closest Point Locator *Feedback the location1 : MATLAB Function  TreatAsAtomicUnit=on
  m->cm : Gain  Gain=100
  xy_cmd : Outport
  closest_point : Outport  Port=2
  distance : Outport  Port=3
  path_i : Outport  Port=4
  heading_cmd : Outport  Port=5
  wires:
  Demux1/1 -> Windowed Closest Point Locator *Feedback the location1/1(x)
  Constant2/1 -> Windowed Closest Point Locator *Feedback the location1/3(x_array)
  Constant3/1 -> Windowed Closest Point Locator *Feedback the location1/4(y_array)
  Constant1/1 -> Mod/2
  Sum/1 -> Mod/1
  Demux1/2 -> Windowed Closest Point Locator *Feedback the location1/2(y)
  Mod/1 -> Bias3/1
  xy/1 -> Demux1/1
  look_ahead_d/1 -> m->cm/1
  m->cm/1 -> Floor/1
  Floor/1 -> Sum/1
  Constant/1 -> Selector1/1
  Selector1/1 -> Mux/1
  Constant4/1 -> Selector2/1
  Mux/1 -> xy_cmd/1
  Selector2/1 -> Mux/2
  Windowed Closest Point Locator *Feedback the location1/2(distance) -> distance/1
  Mux1/1 -> closest_point/1
  Bias1/1 -> Selector3/2, Selector4/2
  Selector4/1 -> Mux1/2
  Constant6/1 -> Selector3/1
  Mod1/1 -> Bias1/1
  Constant7/1 -> Mod1/2
  Constant8/1 -> Selector4/1
  Selector3/1 -> Mux1/1
  Windowed Closest Point Locator *Feedback the location1/1(location) -> Sum/2, path_i/1, Mod1/1, Memory/1
  Bias3/1 -> Selector1/2, Selector5/2, Selector2/2
  Constant9/1 -> Selector5/1
  Selector5/1 -> heading_cmd/1
  Time/1 -> GreaterThan/1
  Constant10/1 -> GreaterThan/2
  Constant5/1 -> Windowed Closest Point Locator *Feedback the location1/5(window)
  Memory/1 -> Windowed Closest Point Locator *Feedback the location1/7(previous_location)
  Constant11/1 -> Manual Switch/2
  Manual Switch/1 -> Windowed Closest Point Locator *Feedback the location1/6(global_search)
  GreaterThan/1 -> Manual Switch/1

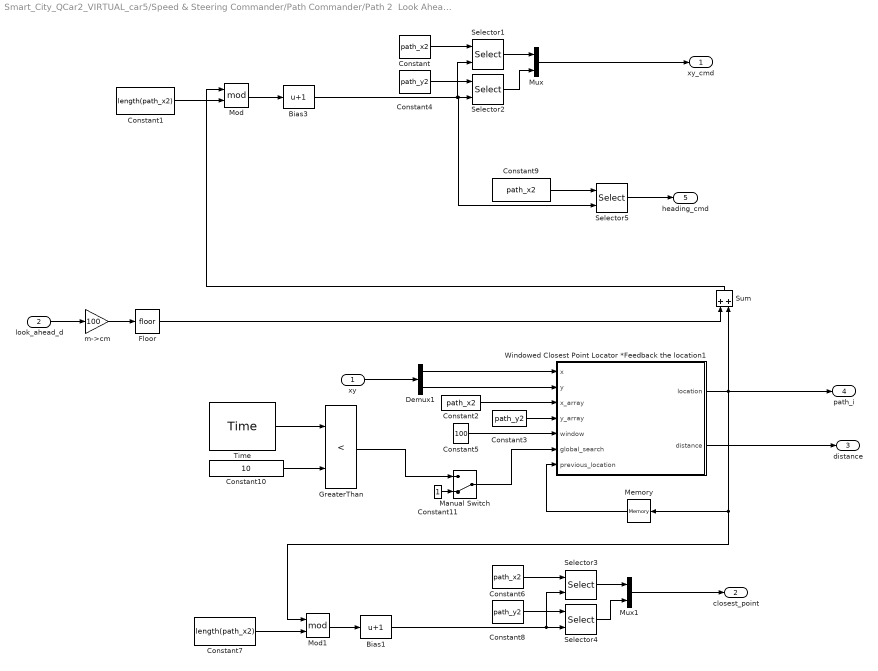
== system Smart_City_QCar2_VIRTUAL_car5/Speed & Steering Commander/Path Commander/Path 2  Look Ahead Generator ==
  xy : Inport
  look_ahead_d : Inport  Port=2
  Bias1 : Bias  Bias=1  SaturateOnIntegerOverflow=off
  Bias3 : Bias  Bias=1  SaturateOnIntegerOverflow=off
  Constant{,2,6,9} (4 alike) : Constant  Value=path_x2
  Constant1 : Constant  Value=length(path_x2)
  Constant10 : Constant  Value=10
  Constant11 : Constant
  Constant3 : Constant  Value=path_y2
  Constant4 : Constant  Value=path_y2
  Constant5 : Constant  Value=100
  Constant7 : Constant  Value=length(path_x2)
  Constant8 : Constant  Value=path_y2
  Demux1 : Demux  Outputs=2
  Floor : Rounding
  GreaterThan : RelationalOperator  Operator=<  OutDataTypeStr=boolean  RndMeth=Simplest  InputSameDT=off
  Manual Switch : ManualSwitch  CurrentSetting=0
  Memory : Memory  InitialCondition=1  InheritSampleTime=on  LinearizeMemory=on  LinearizeAsDelay=on
  Mod : Math  Operator=mod
  Mod1 : Math  Operator=mod
  Mux : Mux  Inputs=2
  Mux1 : Mux  Inputs=2
  Selector{1..5} (5 alike) : Selector  InputPortWidth=length(path_x2)  IndexOptions=Index vector (port)  Indices=[1 3]  OutputSizes=1
  Sum : Sum
  Time : quarc_library/Sources/Time/Time  time_source=Wall clock  sample_time=qc_get_step_size
  Windowed Closest Point Locator *Feedback the location1 : MATLAB Function  TreatAsAtomicUnit=on
  m->cm : Gain  Gain=100
  xy_cmd : Outport
  closest_point : Outport  Port=2
  distance : Outport  Port=3
  path_i : Outport  Port=4
  heading_cmd : Outport  Port=5
  wires:
  Memory/1 -> Windowed Closest Point Locator *Feedback the location1/7(previous_location)
  Constant5/1 -> Windowed Closest Point Locator *Feedback the location1/5(window)
  Selector5/1 -> heading_cmd/1
  Constant9/1 -> Selector5/1
  Bias3/1 -> Selector2/2, Selector5/2, Selector1/2
  Windowed Closest Point Locator *Feedback the location1/1(location) -> Memory/1, Mod1/1, path_i/1, Sum/2
  Constant7/1 -> Mod1/2
  Mod1/1 -> Bias1/1
  Windowed Closest Point Locator *Feedback the location1/2(distance) -> distance/1
  Selector2/1 -> Mux/2
  Mux/1 -> xy_cmd/1
  Constant4/1 -> Selector2/1
  Selector1/1 -> Mux/1
  Constant/1 -> Selector1/1
  Floor/1 -> Sum/1
  m->cm/1 -> Floor/1
  look_ahead_d/1 -> m->cm/1
  xy/1 -> Demux1/1
  Mod/1 -> Bias3/1
  Demux1/2 -> Windowed Closest Point Locator *Feedback the location1/2(y)
  Sum/1 -> Mod/1
  Constant1/1 -> Mod/2
  Constant3/1 -> Windowed Closest Point Locator *Feedback the location1/4(y_array)
  Constant2/1 -> Windowed Closest Point Locator *Feedback the location1/3(x_array)
  Demux1/1 -> Windowed Closest Point Locator *Feedback the location1/1(x)
  Constant8/1 -> Selector4/1
  Selector3/1 -> Mux1/1
  Constant6/1 -> Selector3/1
  Bias1/1 -> Selector3/2, Selector4/2
  Selector4/1 -> Mux1/2
  Mux1/1 -> closest_point/1
  Time/1 -> GreaterThan/1
  Constant10/1 -> GreaterThan/2
  Manual Switch/1 -> Windowed Closest Point Locator *Feedback the location1/6(global_search)
  Constant11/1 -> Manual Switch/2
  GreaterThan/1 -> Manual Switch/1

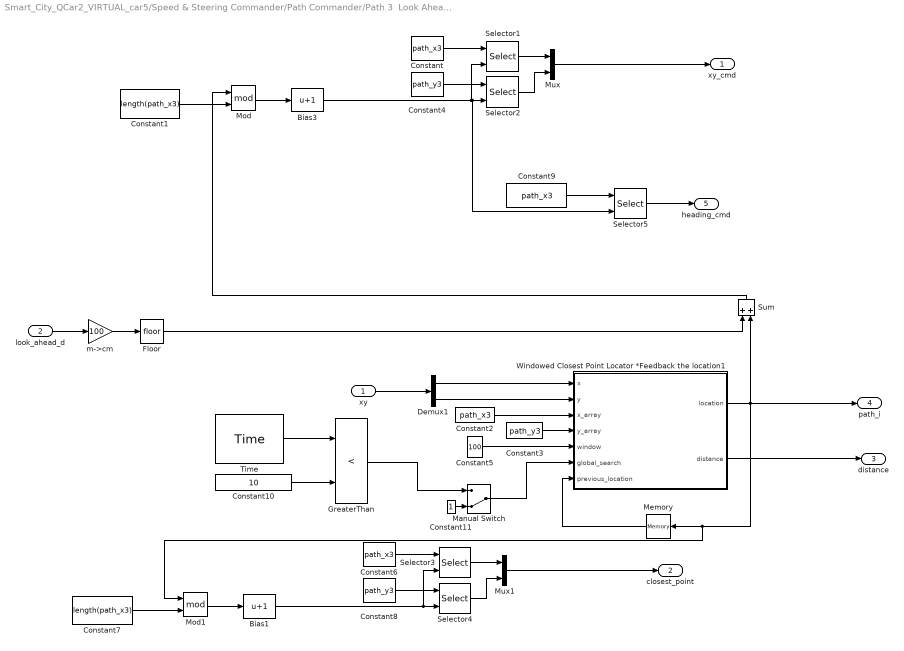
== system Smart_City_QCar2_VIRTUAL_car5/Speed & Steering Commander/Path Commander/Path 3  Look Ahead Generator ==
  xy : Inport
  look_ahead_d : Inport  Port=2
  Bias1 : Bias  Bias=1  SaturateOnIntegerOverflow=off
  Bias3 : Bias  Bias=1  SaturateOnIntegerOverflow=off
  Constant{,2,6,9} (4 alike) : Constant  Value=path_x3
  Constant1 : Constant  Value=length(path_x3)
  Constant10 : Constant  Value=10
  Constant11 : Constant
  Constant3 : Constant  Value=path_y3
  Constant4 : Constant  Value=path_y3
  Constant5 : Constant  Value=100
  Constant7 : Constant  Value=length(path_x3)
  Constant8 : Constant  Value=path_y3
  Demux1 : Demux  Outputs=2
  Floor : Rounding
  GreaterThan : RelationalOperator  Operator=<  OutDataTypeStr=boolean  RndMeth=Simplest  InputSameDT=off
  Manual Switch : ManualSwitch  CurrentSetting=0
  Memory : Memory  InitialCondition=1  InheritSampleTime=on  LinearizeMemory=on  LinearizeAsDelay=on
  Mod : Math  Operator=mod
  Mod1 : Math  Operator=mod
  Mux : Mux  Inputs=2
  Mux1 : Mux  Inputs=2
  Selector{1..5} (5 alike) : Selector  InputPortWidth=length(path_x3)  IndexOptions=Index vector (port)  Indices=[1 3]  OutputSizes=1
  Sum : Sum
  Time : quarc_library/Sources/Time/Time  time_source=Wall clock  sample_time=qc_get_step_size
  Windowed Closest Point Locator *Feedback the location1 : MATLAB Function  TreatAsAtomicUnit=on
  m->cm : Gain  Gain=100
  xy_cmd : Outport
  closest_point : Outport  Port=2
  distance : Outport  Port=3
  path_i : Outport  Port=4
  heading_cmd : Outport  Port=5
  wires:
  Demux1/1 -> Windowed Closest Point Locator *Feedback the location1/1(x)
  Constant2/1 -> Windowed Closest Point Locator *Feedback the location1/3(x_array)
  Constant3/1 -> Windowed Closest Point Locator *Feedback the location1/4(y_array)
  Constant1/1 -> Mod/2
  Sum/1 -> Mod/1
  Demux1/2 -> Windowed Closest Point Locator *Feedback the location1/2(y)
  Mod/1 -> Bias3/1
  xy/1 -> Demux1/1
  look_ahead_d/1 -> m->cm/1
  m->cm/1 -> Floor/1
  Floor/1 -> Sum/1
  Constant/1 -> Selector1/1
  Selector1/1 -> Mux/1
  Constant4/1 -> Selector2/1
  Mux/1 -> xy_cmd/1
  Selector2/1 -> Mux/2
  Windowed Closest Point Locator *Feedback the location1/2(distance) -> distance/1
  Bias3/1 -> Selector1/2, Selector5/2, Selector2/2
  Constant9/1 -> Selector5/1
  Selector5/1 -> heading_cmd/1
  Constant5/1 -> Windowed Closest Point Locator *Feedback the location1/5(window)
  Memory/1 -> Windowed Closest Point Locator *Feedback the location1/7(previous_location)
  Selector4/1 -> Mux1/2
  Selector3/1 -> Mux1/1
  Mux1/1 -> closest_point/1
  Constant8/1 -> Selector4/1
  Windowed Closest Point Locator *Feedback the location1/1(location) -> Sum/2, path_i/1, Mod1/1, Memory/1
  Mod1/1 -> Bias1/1
  Constant6/1 -> Selector3/1
  Constant7/1 -> Mod1/2
  Bias1/1 -> Selector3/2, Selector4/2
  Time/1 -> GreaterThan/1
  Constant10/1 -> GreaterThan/2
  Manual Switch/1 -> Windowed Closest Point Locator *Feedback the location1/6(global_search)
  Constant11/1 -> Manual Switch/2
  GreaterThan/1 -> Manual Switch/1
